simulink model "Simu_Force_Moment_Model_2014"  (R2015a)
settings: Solver=ode45  StartTime=0.0  StopTime=10000  RelTol=1e-3
InitFcn:
  | addpath('../parameters/')
  | aircraft_parameters
  | simulation_parameters
  | sensor_parameters
  | wind_parameters
undefined symbols (not defined in the file or in its folder): drawAircraft, forces_moments, plotmavstatevariables, UAV
libraries: simulink x4
settings Model: CovHtmlReporting=off  CovSFcnEnable=off  Creator=beard  LastModifiedBy=User
settings DataIOCC: SignalLoggingSaveFormat=ModelDataLogs
settings OptimizationCC: ExpressionDepthLimit=2147483647  InitFltsAndDblsToZero=on
settings DebuggingCC: UnderspecifiedInitializationDetection=Classic  MergeDetectMultiDrivingBlocksExec=none  SolverPrmCheckMsg=warning  FcnCallInpInsideContextMsg=EnableAllAsWarning  StateNameClashWarn=warning
settings GRTTargetCC: CombineOutputUpdateFcns=off  GRTInterface=on

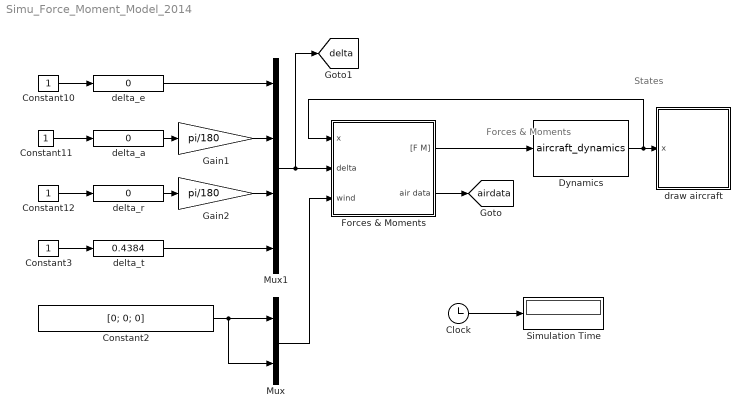
== system Simu_Force_Moment_Model_2014 ==
  note: Forces & Moments
  note: States
  Clock : Clock
  Constant{3,10..12} (4 alike) : Constant
  Constant2 : Constant  Value=[0; 0; 0]
  Dynamics : S-Function  FunctionName=aircraft_dynamics  Parameters=UAV
  Forces & Moments : Subsystem
  Gain1 : Gain  Gain=pi/180
  Gain2 : Gain  Gain=pi/180
  Mux : Mux  Inputs=2
  Mux1 : Mux
  Simulation Time : Display
  delta_a : simulink/Math Operations/Slider Gain  low=-45  gain=0  high=45
  delta_e : simulink/Math Operations/Slider Gain  low=-45  gain=0  high=45
  delta_r : simulink/Math Operations/Slider Gain  low=-45  gain=0  high=45
  delta_t : simulink/Math Operations/Slider Gain  low=0  gain=0.4384  high=1
  draw aircraft : Subsystem
      mask Display: image(imread('tv.jpg'))
  tag scope: airdata=global, delta=global
  wires:
  Constant10/1 -> delta_e/1
  Constant11/1 -> delta_a/1
  Constant12/1 -> delta_r/1
  Dynamics/1 -> Forces & Moments/1(x), draw aircraft/1(x)
  delta_r/1 -> Gain2/1
  delta_a/1 -> Gain1/1
  Constant3/1 -> delta_t/1
  delta_t/1 -> Mux1/4
  Mux1/1 -> [delta], Forces & Moments/2(delta)
  Forces & Moments/1("[F M]") -> Dynamics/1
  Clock/1 -> Simulation Time/1
  Mux/1 -> Forces & Moments/3(wind)
  Forces & Moments/2(air data) -> [airdata]
  delta_e/1 -> Mux1/1
  Gain1/1 -> Mux1/2
  Gain2/1 -> Mux1/3
  Constant2/1 -> Mux/2, Mux/1

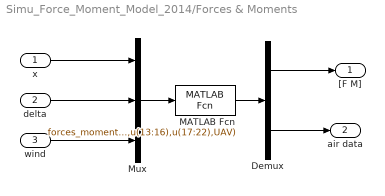
== system Simu_Force_Moment_Model_2014/Forces & Moments ==
  x : Inport
  delta : Inport  Port=2
  wind : Inport  Port=3
  Demux : Demux  Outputs=[6;6]
  MATLAB Fcn : MATLABFcn  MATLABFcn=forces_moments(u(1:12),u(13:16),u(17:22),UAV)  OutputDimensions=12
  Mux : Mux  Inputs=3
  "[F M]" : Outport
  air data : Outport  Port=2
  wires:
  x/1 -> Mux/1
  delta/1 -> Mux/2
  wind/1 -> Mux/3
  MATLAB Fcn/1 -> Demux/1
  Demux/1 -> "[F M]"/1
  Mux/1 -> MATLAB Fcn/1
  Demux/2 -> air data/1

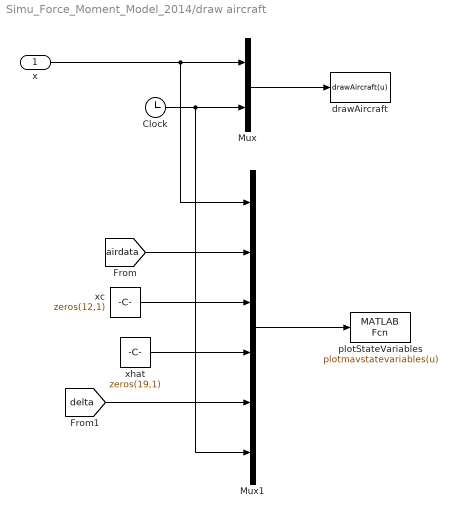
== system Simu_Force_Moment_Model_2014/draw aircraft ==
  x : Inport
  Clock : Clock
  Mux : Mux  Inputs=2
  Mux1 : Mux  Inputs=6
  drawAircraft : MATLABFcn  MATLABFcn=drawAircraft(u)  OutputDimensions=0  SampleTime=0.1
  plotStateVariables : MATLABFcn  MATLABFcn=plotmavstatevariables(u)  OutputDimensions=0  SampleTime=0.1
  xc : Constant  Value=zeros(12,1)
  xhat : Constant  Value=zeros(19,1)
  wires:
  [airdata] -> Mux1/2
  [delta] -> Mux1/5
  xc/1 -> Mux1/3
  xhat/1 -> Mux1/4
  Mux1/1 -> plotStateVariables/1
  Clock/1 -> Mux1/6, Mux/2
  x/1 -> Mux1/1, Mux/1
  Mux/1 -> drawAircraft/1
